simulink model "AKZ_Gen1"  (Simulink 4.00)
settings: Solver=ode23tb  StartTime=0.0  StopTime=5  MaxStep=1e-4  RelTol=1e-3
InitFcn:
  | powericon('psbinitsys',bdroot);
libraries: powerlib2 x10, powerlib_extras x2, simulink_extras x1
settings Model: LastModifiedBy=ieao  BlockReductionOpt=off

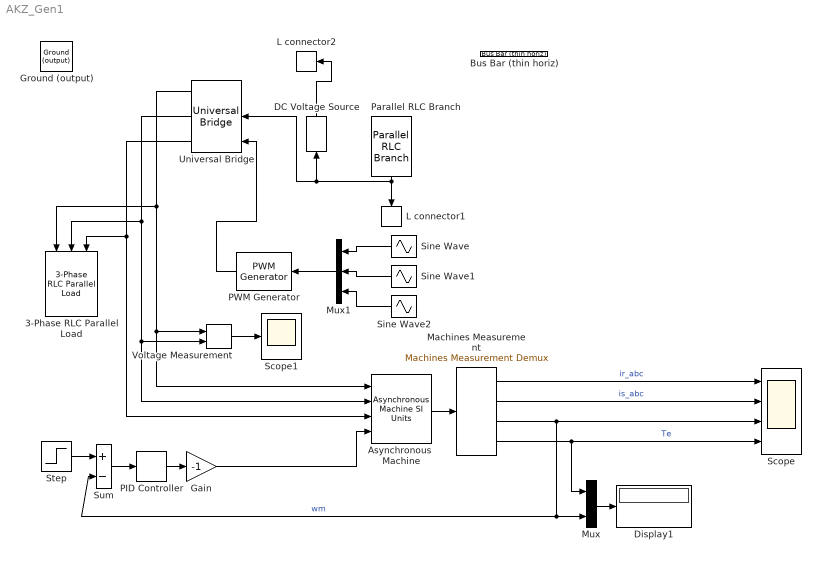
== system AKZ_Gen1 ==
  3-Phase RLC Parallel Load : powerlib_extras/Three-Phase Library/3-Phase RLC Parallel Load  Orientation=down  Vpp=380  fn=50  P3=50e5  QL3=0  QC3=50e5
  "Asynchronous  Machine " : powerlib2/Machines/Asynchronous Machine SI Units  Tag=PoWeRsYsTeMbLoCk  rotType=Squirrel-cage  ctrl=Stationary  x1=[2e5, 380 50 ]  x2="[ 0.435  2.0e-3 ]"  x3="[ 0.00816  2.0e-3 ]"  x4=69.31e-3  x5="[ .89  0  2 ]"  x6="[ 0,0   0,0,0   0,0,0 ]"  PSBOutputType=1110  iounits=1
  Bus Bar (thin horiz) : powerlib2/Connectors/Bus Bar (thin horiz)  Tag=PoWeRsYsTeMbLoCk  Orientation=down  input=0  output=2  PSBOutputType=111111111111111111111111111111111111111111111111111111111111111111111111111111111111
  DC Voltage Source : powerlib2/Electrical Sources/DC Voltage Source  Tag=PoWeRsYsTeMbLoCk  Description=source block  Orientation=up  V=5000  mesure=None  PSBOutputType=1
  Display1 : Display
      settings: Format=short
  Gain : Gain  Gain=-1  Multiplication=Element-wise(K.*u)  SaturateOnIntegerOverflow=on
  Ground (output) : powerlib2/Connectors/Ground (output)  Tag=PoWeRsYsTeMbLoCk  Orientation=up  PSBOutputType=1
  L connector1 : powerlib2/Connectors/L connector  Tag=PoWeRsYsTeMbLoCk  Orientation=left
  L connector2 : powerlib2/Connectors/L connector  Tag=PoWeRsYsTeMbLoCk  Orientation=left
  Machines Measurement : powerlib2/Machines/Machines Measurement Demux  machType=Asynchronous  ssm1=on  ssm2=on  ssm3=on  ssm4=on  ssm5=on  ssm6=on  sm1=on  sm2=on  sm3=on  sm4=on  sm5=on  sm6=on  sm7=on  sm8=on  sm9=on  sm10=on  sm11=on  asm1=off  asm2=on  asm3=off  asm4=off  asm5=on  asm6=off  asm7=off  asm8=off  asm9=on  asm10=on  asm11=off  pmsm1=on  pmsm2=on  pmsm3=on  pmsm4=on  pmsm5=on  pmsm6=on  lastType=1
  Mux : Mux  Inputs=2
      settings: DisplayOption=none
  Mux1 : Mux  Orientation=left  Inputs=3
  PID Controller : simulink_extras/Additional Linear/PID Controller  P=10  I=100  D=0
  PWM Generator : powerlib_extras/Control  Blocks/PWM Generator  Orientation=left  GeneratorMode="3-arm  bridge (6 pulses)"  Fc=1000  Internal=off  mIndex=0.4  Freq=60  Phase=0
  Parallel RLC Branch : powerlib2/Elements/Parallel RLC Branch  Tag=PoWeRsYsTeMbLoCk  Orientation=down  a=100  b=inf  c=1e-4  mesure=None  PSBOutputType=1
  Scope : Scope  NumInputPorts=4
      settings: TimeRange=auto  YMin=-500~-500~70~-600  YMax=400~500~170~100  SaveToWorkspace=off  SaveName=ScopeData  MaxDataPoints=5000
  Scope1 : Scope
      settings: TimeRange=auto  YMin=-1000  YMax=1000  SaveToWorkspace=off  MaxDataPoints=5000
  Sine Wave : Sin  Orientation=left  SineType=Time-based  Amplitude=1  Bias=0  Frequency=314  Phase=-pi/6  Samples=10  SampleTime=0  Offset=0
  Sine Wave1 : Sin  Orientation=left  SineType=Time-based  Amplitude=1  Bias=0  Frequency=314  Phase=-2*pi/3-pi/6  Samples=10  SampleTime=0  Offset=0
  Sine Wave2 : Sin  Orientation=left  SineType=Time-based  Amplitude=1  Bias=0  Frequency=314  Phase=2*pi/3-pi/6  Samples=10  SampleTime=0  Offset=0
  Step : Step  Time=0.05  Before=0  After=160  SampleTime=0
  Sum : Sum  Inputs=+-  SaturateOnIntegerOverflow=on
  Universal Bridge : powerlib2/Power Electronics/Universal Bridge  Tag=PoWeRsYsTeMbLoCk  Orientation=left  arms=3  confi=ABC as output terminals  injcc=1e5  cf=inf  device=IGBT / Diodes  Ron=1e-1  Lon=0  VFs="[  0.8  0.8  ]"  Vf=0  gtoparameters=[ 10e-6 , 20e-6 ]  igbtparameters=[ 1e-6 , 2e-6 ]  mesure=None  PSBOutputType=111
  Voltage Measurement : powerlib2/Measurements/Voltage Measurement  Tag=PoWeRsYsTeMmEaSuReMeNt  PSBOutputType=0  PSBequivalent=1
  wires:
  "Asynchronous  Machine "/1 -> Machines Measurement/1
  Universal Bridge/1 -> "Asynchronous  Machine "/1, Voltage Measurement/1, 3-Phase RLC Parallel Load/1
  Universal Bridge/2 -> "Asynchronous  Machine "/2, Voltage Measurement/2, 3-Phase RLC Parallel Load/2
  Machines Measurement/1 -> Scope/1  "ir_abc"
  Machines Measurement/2 -> Scope/2  "is_abc"
  Machines Measurement/3 -> Mux/2, Sum/2, Scope/3  "wm"
  Machines Measurement/4 -> Mux/1, Scope/4  "Te"
  Mux/1 -> Display1/1
  Step/1 -> Sum/1
  Sum/1 -> PID Controller/1
  PID Controller/1 -> Gain/1
  Gain/1 -> "Asynchronous  Machine "/4
  ? -> Universal Bridge/1, L connector2/Enable
  Parallel RLC Branch/1 -> L connector1/Enable, Universal Bridge/2, DC Voltage Source/1
  ? -> L connector1/1
  Universal Bridge/3 -> "Asynchronous  Machine "/3, 3-Phase RLC Parallel Load/3
  Sine Wave/1 -> Mux1/1
  Sine Wave1/1 -> Mux1/2
  Sine Wave2/1 -> Mux1/3
  PWM Generator/1 -> Universal Bridge/3
  Mux1/1 -> PWM Generator/1
  Voltage Measurement/1 -> Scope1/1
  DC Voltage Source/1 -> L connector2/1
